simulink model "pandoolmakoos"  (R2014a)
settings: Solver=ode45  StartTime=0.0  StopTime=10  RelTol=1e-3
undefined symbols (not defined in the file): g, l, m, mc, x1_0, x2_0
libraries: fuzblock x3
settings Model: Creator=Fifi  LastModifiedBy=Fifi

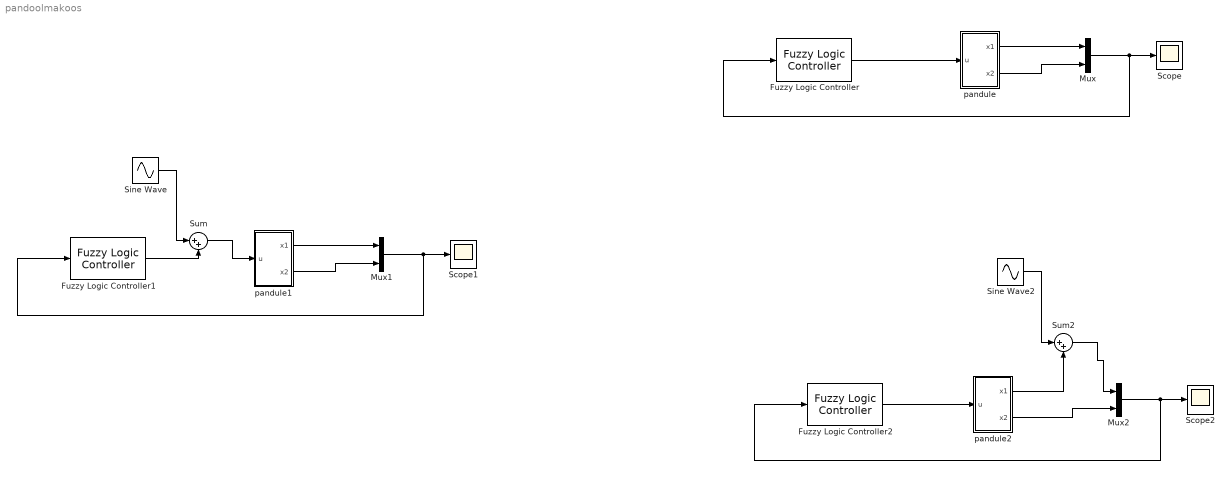
== system pandoolmakoos ==
  Fuzzy Logic Controller : fuzblock/Fuzzy Logic  Controller  fis='pandoolmakoos.fis'
  Fuzzy Logic Controller1 : fuzblock/Fuzzy Logic  Controller  fis='pandoolmakoos.fis'
  Fuzzy Logic Controller2 : fuzblock/Fuzzy Logic  Controller  fis='pandoolmakoos.fis'
  Mux : Mux  Inputs=2
  Mux1 : Mux  Inputs=2
  Mux2 : Mux  Inputs=2
  Scope : Scope
      settings: YMin=-4  YMax=1.75
  Scope1 : Scope
  Scope2 : Scope
      settings: SaveName=ScopeData2
  Sine Wave : Sin  Frequency=5  SampleTime=0
  Sine Wave2 : Sin  Frequency=5  SampleTime=0
  Sum : Sum  Inputs=|++
  Sum2 : Sum  Inputs=|++
  pandule : Subsystem
  pandule1 : Subsystem
  pandule2 : Subsystem
  wires:
  Mux/1 -> Fuzzy Logic Controller/1, Scope/1
  pandule/2(x2) -> Mux/2
  pandule/1(x1) -> Mux/1
  Fuzzy Logic Controller/1 -> pandule/1(u)
  Mux2/1 -> Fuzzy Logic Controller2/1, Scope2/1
  pandule2/2(x2) -> Mux2/2
  Sine Wave2/1 -> Sum2/1
  Sum2/1 -> Mux2/1
  Fuzzy Logic Controller2/1 -> pandule2/1(u)
  pandule2/1(x1) -> Sum2/2
  Mux1/1 -> Fuzzy Logic Controller1/1, Scope1/1
  pandule1/2(x2) -> Mux1/2
  pandule1/1(x1) -> Mux1/1
  Fuzzy Logic Controller1/1 -> Sum/2
  Sine Wave/1 -> Sum/1
  Sum/1 -> pandule1/1(u)

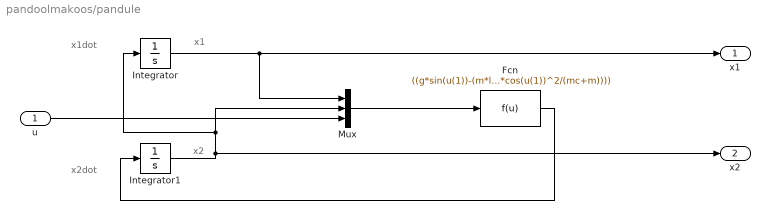
== system pandoolmakoos/pandule ==
  note: x2
  note: x1
  note: x2dot
  note: x1dot
  u : Inport
  Fcn : Fcn  Expr=((g*sin(u(1))-(m*l*u(2)^2*cos(u(1))*sin(u(1))/((mc+m))+cos(u(1))/(mc+m)*u(3))))/(l*(4/3-(m*cos(u(1))^2/(mc+m))))
  Integrator : Integrator  InitialCondition=x1_0
  Integrator1 : Integrator  InitialCondition=x2_0
  Mux : Mux  Inputs=3
  x1 : Outport
  x2 : Outport  Port=2
  wires:
  Integrator/1 -> x1/1, Mux/1
  u/1 -> Mux/3
  Mux/1 -> Fcn/1
  Integrator1/1 -> x2/1, Integrator/1, Mux/2
  Fcn/1 -> Integrator1/1

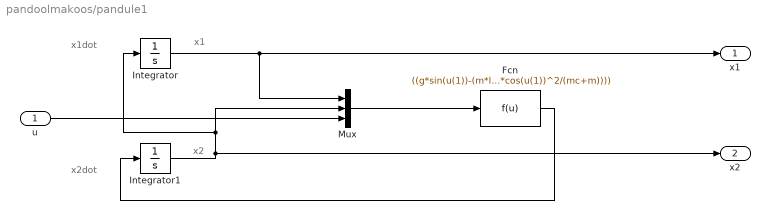
== system pandoolmakoos/pandule1 ==
  note: x2
  note: x1
  note: x2dot
  note: x1dot
  u : Inport
  Fcn : Fcn  Expr=((g*sin(u(1))-(m*l*u(2)^2*cos(u(1))*sin(u(1))/((mc+m))+cos(u(1))/(mc+m)*u(3))))/(l*(4/3-(m*cos(u(1))^2/(mc+m))))
  Integrator : Integrator  InitialCondition=x1_0
  Integrator1 : Integrator  InitialCondition=x2_0
  Mux : Mux  Inputs=3
  x1 : Outport
  x2 : Outport  Port=2
  wires:
  Integrator/1 -> x1/1, Mux/1
  u/1 -> Mux/3
  Mux/1 -> Fcn/1
  Integrator1/1 -> x2/1, Integrator/1, Mux/2
  Fcn/1 -> Integrator1/1

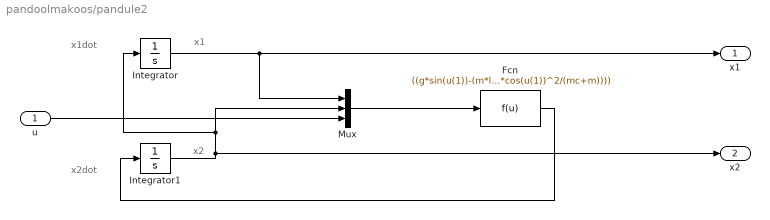
== system pandoolmakoos/pandule2 ==
  note: x2
  note: x1
  note: x2dot
  note: x1dot
  u : Inport
  Fcn : Fcn  Expr=((g*sin(u(1))-(m*l*u(2)^2*cos(u(1))*sin(u(1))/((mc+m))+cos(u(1))/(mc+m)*u(3))))/(l*(4/3-(m*cos(u(1))^2/(mc+m))))
  Integrator : Integrator  InitialCondition=x1_0
  Integrator1 : Integrator  InitialCondition=x2_0
  Mux : Mux  Inputs=3
  x1 : Outport
  x2 : Outport  Port=2
  wires:
  Integrator/1 -> x1/1, Mux/1
  u/1 -> Mux/3
  Mux/1 -> Fcn/1
  Integrator1/1 -> x2/1, Integrator/1, Mux/2
  Fcn/1 -> Integrator1/1
